simulink model "compare_3controller_2016b"  (R2016b)
settings: Solver=ode45  StartTime=0.0  StopTime=150  RelTol=1e-3  EnableMultiTasking=on
PreLoadFcn:
  | mohu=readfis('mohu.fis');
  | lakj=readfis('lakj.fis');
libraries: fuzblock x2, powerlib_extras x1
settings Model: Creator=Administrator  LastModifiedBy=admin
settings SolverCC: ZeroCrossControl=DisableAll
settings DataIOCC: LimitDataPoints=on  SaveFormat=Array  SignalLoggingSaveFormat=ModelDataLogs  SaveOutput=off  SignalLogging=off  DSMLogging=off  SaveTime=off
settings OptimizationCC: ExpressionDepthLimit=2147483647  LifeSpan=inf
settings DebuggingCC: UnderspecifiedInitializationDetection=Classic  MergeDetectMultiDrivingBlocksExec=none  FcnCallInpInsideContextMsg=warning  StateNameClashWarn=warning  SFUnexpectedBacktrackingDiag=warning  SFNoUnconditionalDefaultTransitionDiag=warning  SFExecutionAtInitializationDiag=none
settings HardwareCC: ProdBitPerPointer=32  ProdBitPerSizeT=32  ProdBitPerPtrDiffT=32  ProdLargestAtomicFloat=None  ProdIntDivRoundTo=Undefined  ProdEndianess=Unspecified  ProdWordSize=32  ProdHWDeviceType=32-bit Generic
settings ModelReferenceCC: PropagateSignalLabelsOutOfModel=off
settings GRTTargetCC: TargetLangStandard=C89/C90 (ANSI)  CombineOutputUpdateFcns=off  GRTInterface=on
settings ConfigComp: CovMetricSettings=dw  CovHtmlReporting=on  CovSaveCumulativeToWorkspaceVar=on  CovSaveSingleToWorkspaceVar=on  CovExternalEMLEnable=off

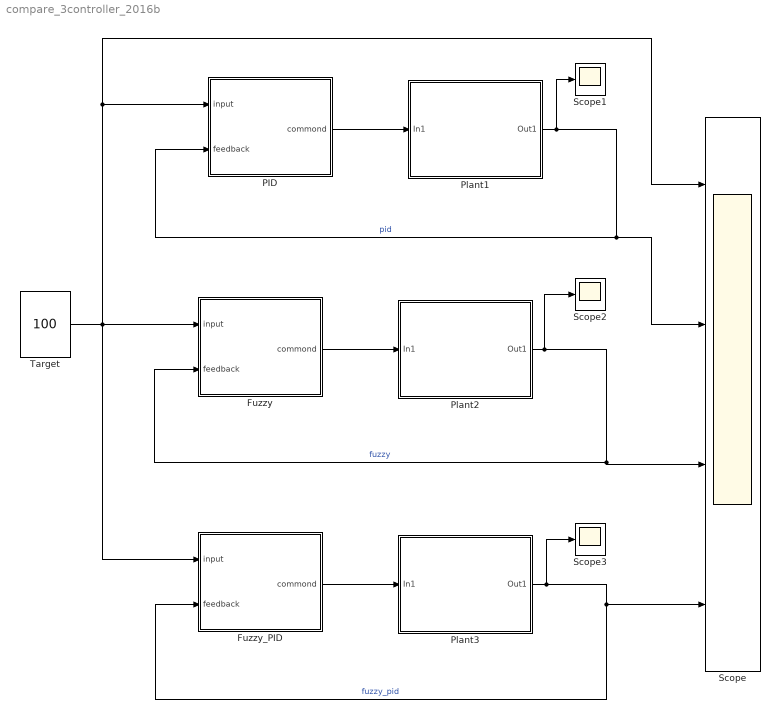
== system compare_3controller_2016b ==
  Fuzzy : Subsystem
  Fuzzy_PID : Subsystem
  PID : Subsystem
  Plant1 : Subsystem
      mask Display: fprintf('Plant')
  Plant2 : Subsystem
      mask Display: fprintf('Plant')
  Plant3 : Subsystem
      mask Display: fprintf('Plant')
  Scope : Scope  NumInputPorts=4
  Scope1 : Scope
  Scope2 : Scope
  Scope3 : Scope
  Target : Constant  Value=100
  wires:
  Target/1 -> Scope/1, PID/1(input), Fuzzy_PID/1(input), Fuzzy/1(input)
  Plant2/1(Out1) -> Scope2/1, Scope/3, Fuzzy/2(feedback)  "fuzzy"
  Fuzzy/1("commond ") -> Plant2/1(In1)
  PID/1("commond ") -> Plant1/1(In1)
  Plant3/1(Out1) -> Scope3/1, Scope/4, Fuzzy_PID/2(feedback)  "fuzzy_pid"
  Fuzzy_PID/1("commond ") -> Plant3/1(In1)
  Plant1/1(Out1) -> Scope1/1, Scope/2, PID/2(feedback)  "pid"

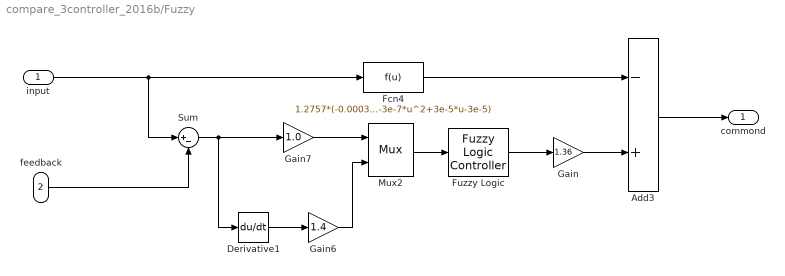
== system compare_3controller_2016b/Fuzzy ==
  input : Inport
  feedback : Inport  Port=2
  Add3 : Sum  Inputs=-+
  Derivative1 : Derivative
  Fcn4 : Fcn  Expr=1.2757*(-0.0003*u^2+0.1401*u-0.1236)+2.4164e-6*(10278*u-35310)-3.9398e-4*(-0.0003*u^2+0.1401*u-0.1236)^2-1.9519e-15*(10278*u-35310)^2+1.0422e4*(-1e-12*u^4+1e-9*u^3-3e-7*u^2+3e-5*u-3e-5)
  "Fuzzy Logic " : fuzblock/Fuzzy Logic  Controller  fis=lakj
  Gain : Gain  Gain=1.36
  Gain6 : Gain  Gain=1.4
  Gain7 : Gain  Gain=1.0
  Mux2 : Mux  Inputs=2
  Sum : Sum  Inputs=|+-
  "commond " : Outport
  wires:
  feedback/1 -> Sum/2
  input/1 -> Sum/1, Fcn4/1
  Fcn4/1 -> Add3/1
  Add3/1 -> "commond "/1
  Derivative1/1 -> Gain6/1
  Gain6/1 -> Mux2/2
  "Fuzzy Logic "/1 -> Gain/1
  Gain7/1 -> Mux2/1
  Mux2/1 -> "Fuzzy Logic "/1
  Sum/1 -> Derivative1/1, Gain7/1
  Gain/1 -> Add3/2

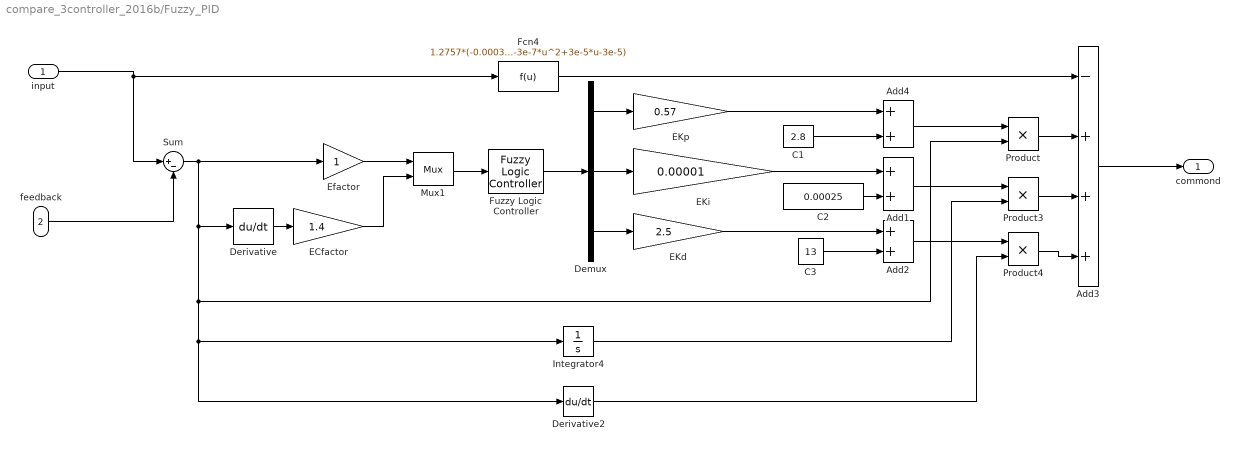
== system compare_3controller_2016b/Fuzzy_PID ==
  input : Inport
  feedback : Inport  Port=2
  Add1 : Sum
  Add2 : Sum
  Add3 : Sum  Inputs=-+++
  Add4 : Sum
  C1 : Constant  Value=2.8
  C2 : Constant  Value=0.00025
  C3 : Constant  Value=13
  Demux : Demux  Outputs=3
  Derivative : Derivative
  Derivative2 : Derivative
  ECfactor : Gain  Gain=1.4
  EKd : Gain  Gain=2.5
  EKi : Gain  Gain=0.00001
  EKp : Gain  Gain=0.57
  Efactor : Gain
  Fcn4 : Fcn  Expr=1.2757*(-0.0003*u^2+0.1401*u-0.1236)+2.4164e-6*(10278*u-35310)-3.9398e-4*(-0.0003*u^2+0.1401*u-0.1236)^2-1.9519e-15*(10278*u-35310)^2+1.0422e4*(-1e-12*u^4+1e-9*u^3-3e-7*u^2+3e-5*u-3e-5)
  Fuzzy Logic Controller : fuzblock/Fuzzy Logic  Controller  fis=mohu
  Integrator4 : Integrator
  Mux1 : Mux  Inputs=2
  Product : Product  RndMeth=Zero
  Product3 : Product  RndMeth=Zero
  Product4 : Product  RndMeth=Zero
  Sum : Sum  Inputs=|+-
  "commond " : Outport
  wires:
  feedback/1 -> Sum/2
  Sum/1 -> Product/2, Integrator4/1, Derivative2/1, Derivative/1, Efactor/1
  ECfactor/1 -> Mux1/2
  Add1/1 -> Product3/1
  Demux/3 -> EKd/1
  Product4/1 -> Add3/4
  EKi/1 -> Add1/1
  input/1 -> Sum/1, Fcn4/1
  Demux/2 -> EKi/1
  Fcn4/1 -> Add3/1
  Add2/1 -> Product4/1
  Add4/1 -> Product/1
  EKp/1 -> Add4/1
  Product3/1 -> Add3/3
  Efactor/1 -> Mux1/1
  EKd/1 -> Add2/1
  Integrator4/1 -> Product3/2
  Derivative/1 -> ECfactor/1
  Product/1 -> Add3/2
  Derivative2/1 -> Product4/2
  Demux/1 -> EKp/1
  C1/1 -> Add4/2
  C2/1 -> Add1/2
  C3/1 -> Add2/2
  Fuzzy Logic Controller/1 -> Demux/1
  Mux1/1 -> Fuzzy Logic Controller/1
  Add3/1 -> "commond "/1

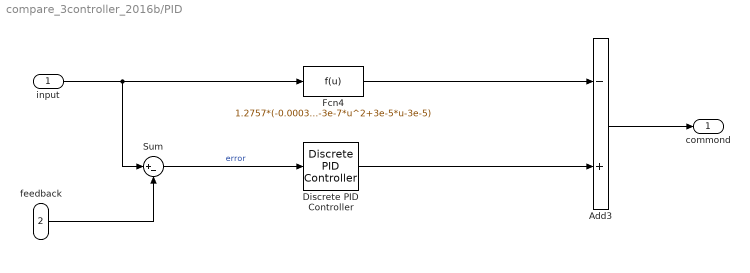
== system compare_3controller_2016b/PID ==
  input : Inport
  feedback : Inport  Port=2
  Add3 : Sum  Inputs=-+
  Discrete PID Controller : powerlib_extras/Discrete  Control Blocks/Discrete PID Controller  Kp=2.8  Ki=0.00025  Kd=13  TcD=1  Par_Limits=[100 -100]  Init=0  Ts=0.5
  Fcn4 : Fcn  Expr=1.2757*(-0.0003*u^2+0.1401*u-0.1236)+2.4164e-6*(10278*u-35310)-3.9398e-4*(-0.0003*u^2+0.1401*u-0.1236)^2-1.9519e-15*(10278*u-35310)^2+1.0422e4*(-1e-12*u^4+1e-9*u^3-3e-7*u^2+3e-5*u-3e-5)
  Sum : Sum  Inputs=|+-
  "commond " : Outport
  wires:
  feedback/1 -> Sum/2
  input/1 -> Sum/1, Fcn4/1
  Fcn4/1 -> Add3/1
  Add3/1 -> "commond "/1
  Sum/1 -> Discrete PID Controller/1  "error"
  Discrete PID Controller/1 -> Add3/2

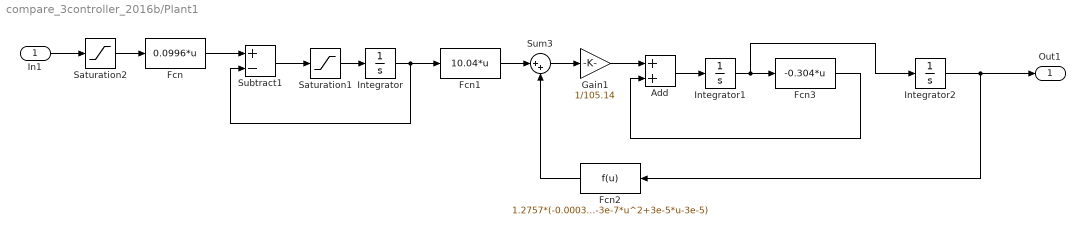
== system compare_3controller_2016b/Plant1 ==
  In1 : Inport
  Add : Sum
  Fcn : Fcn  Expr=0.0996*u
  Fcn1 : Fcn  Expr=10.04*u
  Fcn2 : Fcn  Expr=1.2757*(-0.0003*u^2+0.1401*u-0.1236)+2.4164e-6*(10278*u-35310)-3.9398e-4*(-0.0003*u^2+0.1401*u-0.1236)^2-1.9519e-15*(10278*u-35310)^2+1.0422e4*(-1e-12*u^4+1e-9*u^3-3e-7*u^2+3e-5*u-3e-5)
  Fcn3 : Fcn  Expr=-0.304*u
  Gain1 : Gain  Gain=1/105.14
  Integrator : Integrator
  Integrator1 : Integrator
  Integrator2 : Integrator  InitialCondition=90
  Saturation1 : Saturate  UpperLimit=0.167  LowerLimit=-0.167
  Saturation2 : Saturate  UpperLimit=80.36  LowerLimit=-80.36
  Subtract1 : Sum  Inputs=+-
  Sum3 : Sum  Inputs=|++
  Out1 : Outport
  wires:
  Fcn/1 -> Subtract1/1
  Subtract1/1 -> Saturation1/1
  Saturation1/1 -> Integrator/1
  Integrator/1 -> Subtract1/2, Fcn1/1
  Add/1 -> Integrator1/1
  Integrator1/1 -> Fcn3/1, Integrator2/1
  Gain1/1 -> Add/1
  Sum3/1 -> Gain1/1
  Fcn1/1 -> Sum3/1
  Fcn2/1 -> Sum3/2
  Saturation2/1 -> Fcn/1
  Fcn3/1 -> Add/2
  Integrator2/1 -> Fcn2/1, Out1/1
  In1/1 -> Saturation2/1

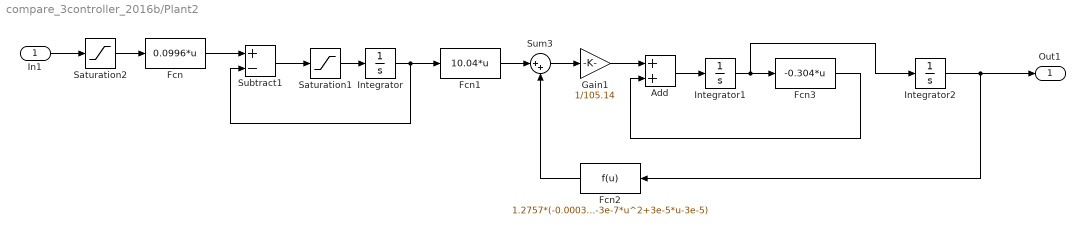
== system compare_3controller_2016b/Plant2 ==
  In1 : Inport
  Add : Sum
  Fcn : Fcn  Expr=0.0996*u
  Fcn1 : Fcn  Expr=10.04*u
  Fcn2 : Fcn  Expr=1.2757*(-0.0003*u^2+0.1401*u-0.1236)+2.4164e-6*(10278*u-35310)-3.9398e-4*(-0.0003*u^2+0.1401*u-0.1236)^2-1.9519e-15*(10278*u-35310)^2+1.0422e4*(-1e-12*u^4+1e-9*u^3-3e-7*u^2+3e-5*u-3e-5)
  Fcn3 : Fcn  Expr=-0.304*u
  Gain1 : Gain  Gain=1/105.14
  Integrator : Integrator
  Integrator1 : Integrator
  Integrator2 : Integrator  InitialCondition=90
  Saturation1 : Saturate  UpperLimit=0.167  LowerLimit=-0.167
  Saturation2 : Saturate  UpperLimit=80.36  LowerLimit=-80.36
  Subtract1 : Sum  Inputs=+-
  Sum3 : Sum  Inputs=|++
  Out1 : Outport
  wires:
  Integrator2/1 -> Fcn2/1, Out1/1
  Integrator/1 -> Subtract1/2, Fcn1/1
  Fcn3/1 -> Add/2
  Saturation1/1 -> Integrator/1
  Integrator1/1 -> Fcn3/1, Integrator2/1
  Saturation2/1 -> Fcn/1
  Fcn1/1 -> Sum3/1
  Add/1 -> Integrator1/1
  In1/1 -> Saturation2/1
  Fcn2/1 -> Sum3/2
  Gain1/1 -> Add/1
  Fcn/1 -> Subtract1/1
  Subtract1/1 -> Saturation1/1
  Sum3/1 -> Gain1/1

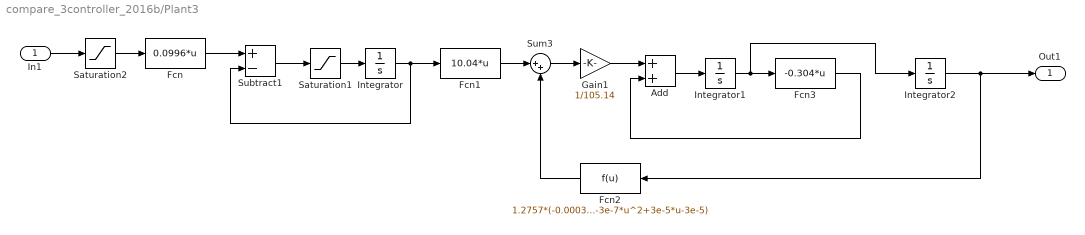
== system compare_3controller_2016b/Plant3 ==
  In1 : Inport
  Add : Sum
  Fcn : Fcn  Expr=0.0996*u
  Fcn1 : Fcn  Expr=10.04*u
  Fcn2 : Fcn  Expr=1.2757*(-0.0003*u^2+0.1401*u-0.1236)+2.4164e-6*(10278*u-35310)-3.9398e-4*(-0.0003*u^2+0.1401*u-0.1236)^2-1.9519e-15*(10278*u-35310)^2+1.0422e4*(-1e-12*u^4+1e-9*u^3-3e-7*u^2+3e-5*u-3e-5)
  Fcn3 : Fcn  Expr=-0.304*u
  Gain1 : Gain  Gain=1/105.14
  Integrator : Integrator
  Integrator1 : Integrator
  Integrator2 : Integrator  InitialCondition=90
  Saturation1 : Saturate  UpperLimit=0.167  LowerLimit=-0.167
  Saturation2 : Saturate  UpperLimit=80.36  LowerLimit=-80.36
  Subtract1 : Sum  Inputs=+-
  Sum3 : Sum  Inputs=|++
  Out1 : Outport
  wires:
  Integrator2/1 -> Fcn2/1, Out1/1
  Integrator/1 -> Subtract1/2, Fcn1/1
  Fcn3/1 -> Add/2
  Saturation1/1 -> Integrator/1
  Integrator1/1 -> Fcn3/1, Integrator2/1
  Saturation2/1 -> Fcn/1
  Fcn1/1 -> Sum3/1
  Add/1 -> Integrator1/1
  In1/1 -> Saturation2/1
  Fcn2/1 -> Sum3/2
  Gain1/1 -> Add/1
  Fcn/1 -> Subtract1/1
  Subtract1/1 -> Saturation1/1
  Sum3/1 -> Gain1/1
